simulink model "sampleTimeCount"  (R2024b)
settings: Solver=FixedStepAuto  StartTime=0.0  StopTime=50  FixedStep=1  RelTol=1e-3
libraries: simulink x1
settings Model: Creator=z004f2se  LastModifiedBy=z004f2se

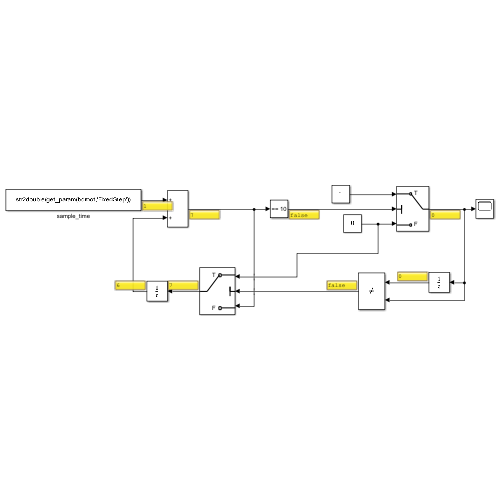
[thumbnail: Simulink's stored preview of the top-level diagram]
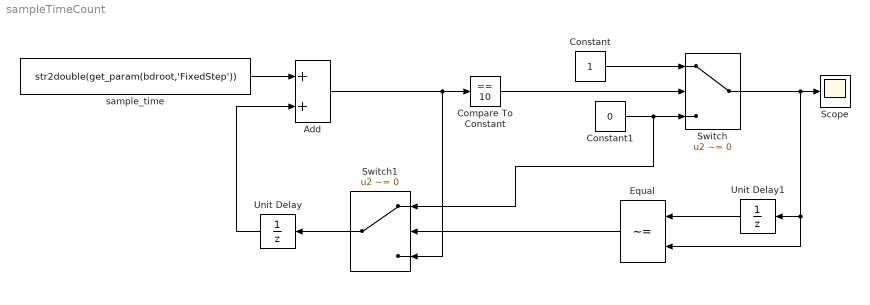
== system sampleTimeCount ==
  Add : Sum
  Compare To Constant : simulink/Logic and Bit Operations/Compare To Constant  relop===  const=10  OutDataTypeStr=boolean
  Constant : Constant
  Constant1 : Constant  Value=0
  Equal : RelationalOperator  Operator=~=  OutDataTypeStr=boolean  RndMeth=Simplest  InputSameDT=off
  Scope : Scope
  Switch : Switch  Criteria=u2 ~= 0  Threshold=10  SaturateOnIntegerOverflow=off  InputSameDT=off
  Switch1 : Switch  Criteria=u2 ~= 0  SaturateOnIntegerOverflow=off  InputSameDT=off
  Unit Delay : UnitDelay  SampleTime=-1  HasFrameUpgradeWarning=on
  Unit Delay1 : UnitDelay  SampleTime=-1  HasFrameUpgradeWarning=on
  sample_time : Constant  Value=str2double(get_param(bdroot,'FixedStep'))
  wires:
  sample_time/1 -> Add/1
  Add/1 -> Switch1/3, Compare To Constant/1
  Constant1/1 -> Switch1/1, Switch/3
  Constant/1 -> Switch/1
  Compare To Constant/1 -> Switch/2
  Switch/1 -> Equal/2, Unit Delay1/1, Scope/1
  Unit Delay1/1 -> Equal/1
  Equal/1 -> Switch1/2
  Switch1/1 -> Unit Delay/1
  Unit Delay/1 -> Add/2
